simulink model "BBK_client_2012b"  (R2012b)
settings: Solver=ode3  StartTime=0.0  StopTime=Inf  FixedStep=base_dT  MaxStep=0.01  RelTol=1e-3
values from neighbouring files (symbols this model uses):
  base_dT = Simulink.Parameter    [InternetBBKInit.m]
libraries: simulink x1
settings Model: Creator=akshart  LastModifiedBy=Hcn
settings DataIOCC: SignalLoggingSaveFormat=ModelDataLogs
settings OptimizationCC: InitFltsAndDblsToZero=on
settings DebuggingCC: FcnCallInpInsideContextMsg=EnableAllAsWarning  FrameProcessingCompatibilityMsg=error
settings CodeAppCC: CustomSymbolStrType=$N$R$M_T
settings GRTTargetCC: CodeReplacementLibrary=C89/C90 (ANSI)  CombineOutputUpdateFcns=off  GRTInterface=on

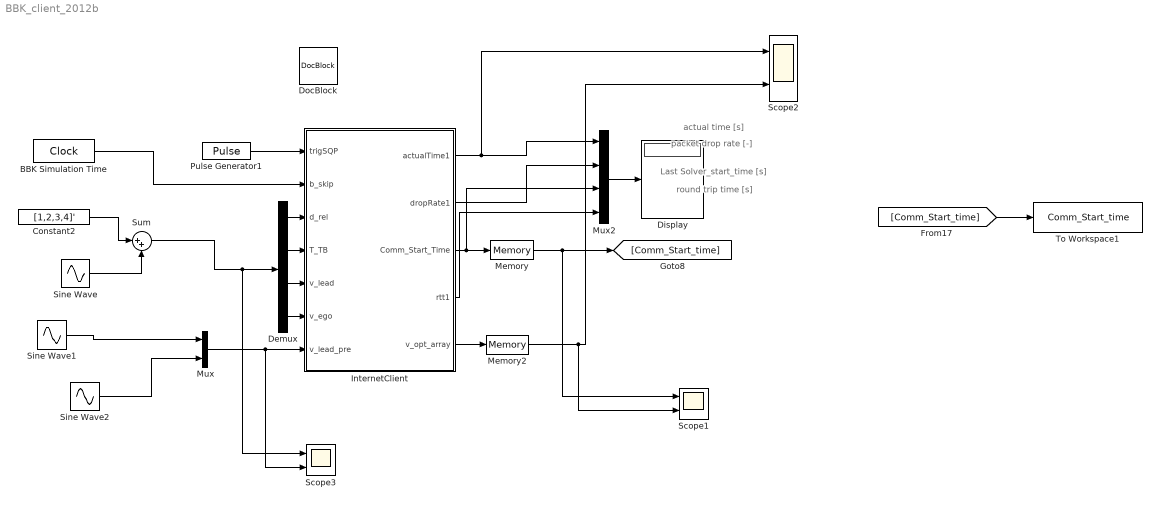
== system BBK_client_2012b ==
  note: actual time [s]
  note: packet drop rate [-]
  note: Last Solver_start_time [s]
  note: round trip time [s]
  BBK Simulation Time : DigitalClock  SampleTime=base_dT
  Constant2 : Constant  Value=[1,2,3,4]'
  Demux : Demux
  Display : Display
  DocBlock : simulink/Model-Wide Utilities/DocBlock  DocumentType=Text
      content=|
      | Type your documentation here
      |
      | Time                Version Note
      | 101019T1524         Change Ne profile to be slower by changing Driver_Rsl.
      | 101519T2324         Change torque converter torque_ratio in deceleration to make decel Ne fit better.
      | 102219T1600         Integrate solver in Intern_v11 with follower model.
      | 102419T1340         Replace the follower model with 102219T1630 follower model.
      |                     change "off-delay" block to make it run-able in function-call-subsys.
      |                     change multiple continuous solver/integrator to discrete time.
      |                     change multiple delay to discrete time.
      |                     solve "computation loop" problem.
      |                     remove global data store "solver_exec_ctr".
      | 102519T1650         Change the P and I gain for driver_model to be doubled.
      |                     And then changed back, because with the old P and I gains, fuel matches better with data.
      |                     To solve the Ne and speed tracking problem, saturate Ne integrator by 600 and 3400.
      | 102819T1200         Ddd saturation to match idle fuel, only affect fuel consumption number, do not affect driveline.
      |                     Change GearShifting model to have upshift limits: 1600,1800rpm.
      |                     Second bag when vehicle at move (MD.VESP_mph/2.236>=1.5m/s) fuel consumption:
      |                     data fuel at move is -- 764.1621 [g]
      |                     simulink fuel at move is -- 776.5815 [g], +1.63% error.
      | 102819T2340         Change the "follow vehicle1"-->"gain"0.44 place to before acce_filter.
      |                     Previously "filtered_acce" has unit mph/s...
      |                     Change "follow vehicle1"-->"time constant" from 0.5s to 2s.
      |                     data fuel at move is -- 764.5319 [g]
      |                     simulink fuel at move is -- 771.5589 [g], +1.0% error.
      | 102919T1500         -Add substraction for E2C_tiSolverPeriod_C. Because stateflow will add 1 base_dT step.
      |                     Use SendDemand on "E2C_model" subsys to avoid delay introduced by solver_end_time.
      |                     Add function-call subsystem in "E2C_model/solver".
      |                     This way will syncronize with v_ego_array output, and
      |                     update once new optimal v_ego_array is available.
      |                     -"E2C_model/solver/Send  V_demand", add "Matlab Function1" to
      |                     use previous optimal speed as current target speed.
      | 102919T1700         -In previous version, used delayed(v_opt)(1) as previous optimal speed.
      |                     But should be using v_opt(solver_start-delayed(solver_start) ).
      |                     Modified in this version.
      |                     Note: based on solver_start_time to update v_opt_array.
      |                     If solver starts base_dT(s) after solver ends, then correct.
      | 102919T2100         -In previous version, used delayed(v_opt)(1) as previous optimal speed.
      |                     But should be using v_opt(solver_start-delayed(solver_start) ).
      |                     -Use solver_end_time to update v_opt_array.
      | 103119T1400         -Moved leader system out of E2C
      |                     Put leader subsys and Follower subsystem into one function-call system.
      |                     -Compared results from mpcqpsolver and quadprog, final traces are extremely similar. see
      |                     PlatoonModel_Chunan_2016b_102919Txxxx_19_10_31_14_48,PlatoonModel_Chunan_2016b_102919Txxxx_19_10_31_16_22.
      |                     mpcqpsolver is much faster than quadprog.
      | 110519T1100         -in E2C_model, add option for using triditional ACC.
      |                     Add vars b_use_acc,c_acc_hdw.
      |                     changed .m file for setting parameters.
      | 111119T1200         -in E2C_model, add condition for if t_>t_startsimulation.
      |                     only start after 498s.
      |                     -In subsys, change Driver_TuneG1,Driver_TuneG2 to be calibration vars.
      |                     -make V_Opt_Array_modify to be base_dT_delayed(previous V_Opt_Array_modify). Avoid jumps when v_opt updates.
      |                     -PARS.Driver_TuneG1 = 0.015*16;PARS.Driver_TuneG2 = 5;
      |                     with w=0, much smoother optimal speed than before.
      | 111919T1000         -Dyno subsystem change maps for calculating T_TB.
      | 112119T1155         -Add "ToWorkspace" nodes for TTBego, and solver outputs.
      | Client_112619T1415  -Created from PlatoonModel_Chunan_2016b_112119T1155 and InternetClient_112619T1300.
      |                     -Contains the whole vehicle model.
      |                     -Set up memory for CommOut_V_Opt_Array to align change for CommOut_V_Opt_Array and Comm_Start_Time.
      | Solver_112619T1415  -Created.
      |                     -Add semicolon in state flow to avoid printing intermediate variables.
      | C/S_122019T1424     -Add to resolve rtt issue. Not very useful on full model.:
      |                             while (myIns.simTime > timeNow*1)
      |                          {
      |                              QueryPerformanceCounter(&LItNow);
      |                              timeNow = ((double)(LItNow.QuadPart - G.LIstartTime.QuadPart)) / ((double)(G.LIticksPerSecond.QuadPart)) ;
      |                          }
      | %%%%%%%%%%%%%%%%%%%%%%%%%%%%%%%%%%%%%%%%%%%%%%%%%%%%%%%%%%%%%%%%%%%%%%%%%%
      | %                        3-computer setup                                %
      | %%%%%%%%%%%%%%%%%%%%%%%%%%%%%%%%%%%%%%%%%%%%%%%%%%%%%%%%%%%%%%%%%%%%%%%%%%
      | BBK_01022020T1343
      |                     -Create simulink block.
      |                     -Create "InternetBBKInit.m" file for initialization.
  InternetClient : Subsystem  mask(20-sim 4.6 S-Function block){}
      mask help:
      | This block is generated by the 20-sim Matlab Code Generator.
      |
      | * look under the mask to get information on the ports
      | * press Help for more detailed information
      | * the parameters of this block are:
      mask Help:
      | This block is generated by the 20-sim Matlab Code Generator<br>
      | The block parameters are:<br><blockquote></blockquote>
      | Generated at:<br>
      | <blockquote><b>date:  </b>June 14, 2017<br>
      | <b>time:  </b>4:16:43 PM<br></blockquote>
      | From the following 20-sim model:<br>
      | <blockquote><b>submodel:  </b>InternetServer<br>
      | <b>model:  </b>export to Simulink - UM<br>
      | <b>file:  </b>C:\Users\Tulga Ersal\Desktop\For Xueru\export to Simulink - UM.emx<br>
      | <b>experiment:  </b>C:\Users\Tulga Ersal\Desktop\For Xueru\export to Simulink - UM.emx<br></blockquote>
      | Using the following 20-sim license:<br>
      | <blockquote><b>user:  </b>The University of Michigan<br>
      | <b>from:  </b>20-sim 4.6 Student License<br>
      | <b>build: </b>4.6.1.6898<br></blockquote>
  Memory : Memory  InheritSampleTime=on  LinearizeAsDelay=on
  Memory2 : Memory  X0=zeros(2,1)  InheritSampleTime=on  LinearizeAsDelay=on
  Mux : Mux  Inputs=2
  Mux2 : Mux
  Pulse Generator1 : DiscretePulseGenerator  PulseType=Time based  Period=1  PulseWidth=20  SampleTime=base_dT
  Scope1 : Scope  NumInputPorts=2
      settings: TimeRange=auto  MaxDataPoints=5000  SaveToWorkspace=off  YMin=-0.25~-0.5  YMax=2.25~4.5  SampleTime=-1
  Scope2 : Scope  NumInputPorts=2
      settings: TimeRange=auto  MaxDataPoints=5000  SaveToWorkspace=off  YMin=-3.575~-5  YMax=32.175~5  SampleTime=-1
  Scope3 : Scope  NumInputPorts=2
      settings: TimeRange=auto  MaxDataPoints=5000  SaveToWorkspace=off  SaveName=ScopeData2  YMin=-1.71028~-1.71028  YMax=15.39249~15.39249  SampleTime=-1
  Sine Wave : Sin  SampleTime=0
  Sine Wave1 : Sin  Amplitude=2  SampleTime=0
  Sine Wave2 : Sin  Amplitude=4  Frequency=2  SampleTime=0
  Sum : Sum  Inputs=|++
  To Workspace1 : ToWorkspace  VariableName=Comm_Start_time  SaveFormat=Structure With Time  SampleTime=-1
  wires:
  Constant2/1 -> Sum/1
  InternetClient/3(Comm_Start_Time) -> Mux2/3, Memory/1
  Memory/1 -> Scope1/1, [Comm_Start_time]
  InternetClient/5(v_opt_array) -> Memory2/1
  Pulse Generator1/1 -> InternetClient/1(trigSQP)
  InternetClient/1(actualTime1) -> Scope2/1, Mux2/1
  InternetClient/2(dropRate1) -> Mux2/2
  InternetClient/4(rtt1) -> Mux2/4
  Mux2/1 -> Display/1
  [Comm_Start_time] -> To Workspace1/1
  Memory2/1 -> Scope1/2, Scope2/2
  BBK Simulation Time/1 -> InternetClient/2(b_skip)
  Mux/1 -> Scope3/2, InternetClient/7(v_lead_pre)
  Sine Wave/1 -> Sum/2
  Demux/1 -> InternetClient/3(d_rel)
  Demux/2 -> InternetClient/4(T_TB)
  Demux/3 -> InternetClient/5(v_lead)
  Demux/4 -> InternetClient/6(v_ego)
  Sum/1 -> Scope3/1, Demux/1
  Sine Wave2/1 -> Mux/2
  Sine Wave1/1 -> Mux/1

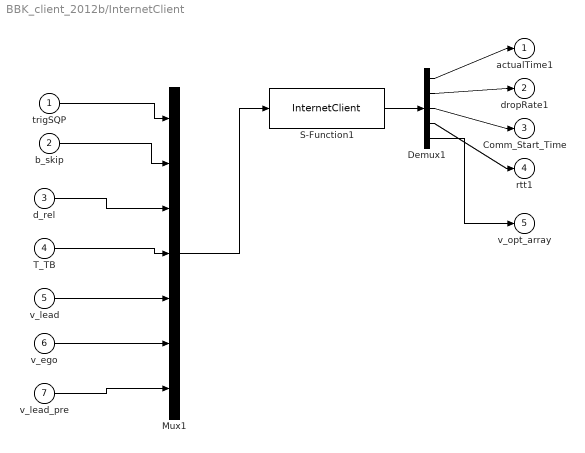
== system BBK_client_2012b/InternetClient ==
  trigSQP : Inport
  b_skip : Inport  Port=2
  d_rel : Inport  Port=3
  T_TB : Inport  Port=4
  v_lead : Inport  Port=5
  v_ego : Inport  Port=6
  v_lead_pre : Inport  Port=7
  Demux1 : Demux  Outputs=[1 1 1 1 2 ]
  Mux1 : Mux  Inputs=[1 1 1 1 1 1 2 ]
  S-Function1 : S-Function  FunctionName=InternetClient  SFunctionDeploymentMode=off  EnableBusSupport=off
  actualTime1 : Outport
  dropRate1 : Outport  Port=2
  Comm_Start_Time : Outport  Port=3
  rtt1 : Outport  Port=4
  v_opt_array : Outport  Port=5
  wires:
  Demux1/1 -> actualTime1/1
  Demux1/2 -> dropRate1/1
  Demux1/3 -> Comm_Start_Time/1
  Demux1/4 -> rtt1/1
  S-Function1/1 -> Demux1/1
  trigSQP/1 -> Mux1/1
  b_skip/1 -> Mux1/2
  Mux1/1 -> S-Function1/1
  T_TB/1 -> Mux1/4
  d_rel/1 -> Mux1/3
  v_lead/1 -> Mux1/5
  v_ego/1 -> Mux1/6
  v_lead_pre/1 -> Mux1/7
  Demux1/5 -> v_opt_array/1
